simulink library "sm_wing_landing_gear_lib"  (R2015a)
settings: Solver=ode45  StartTime=0.0  StopTime=10.0  RelTol=1e-3
undefined symbols (not defined in the file): dgrey, rho_alum, X, Y, Z
libraries: sm_lib x126, sm_wing_landing_gear_lib x1
(part 1 of 4)
Description:
  | Copyright 2008-2015 The MathWorks, Inc.
settings Model: Creator=MathWorks  LastModifiedBy=batserve
settings DataIOCC: SignalLoggingSaveFormat=ModelDataLogs
settings OptimizationCC: ExpressionDepthLimit=2147483647
settings DebuggingCC: UnderspecifiedInitializationDetection=Classic  MergeDetectMultiDrivingBlocksExec=none  SolverPrmCheckMsg=warning  FcnCallInpInsideContextMsg=EnableAllAsWarning  StateNameClashWarn=warning

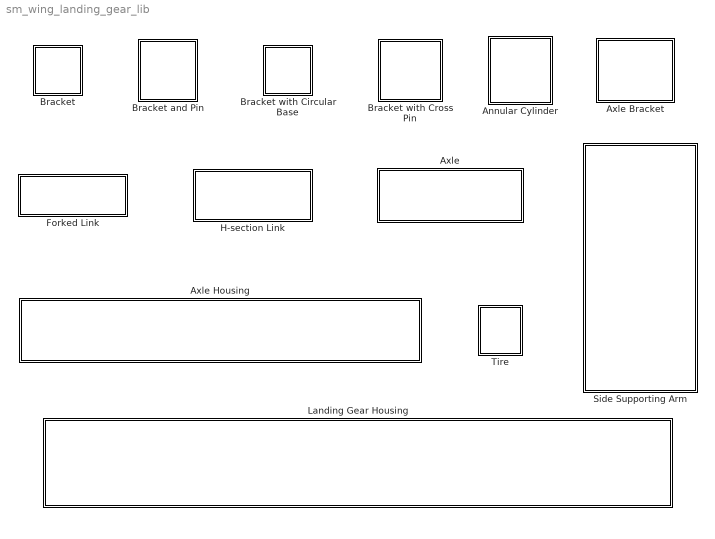
== system sm_wing_landing_gear_lib ==
  Annular Cylinder : Subsystem  mask(Annular Cylinder){Ro=10, Ri=5, L=1, rho=1000, clr=[0.5 0.5 0.5], opc=1}
      mask prompts: Ro "Cylinder outer radius (cm)"; Ri "Cylinder inner radius (cm)"; L "Cylinder length (cm)"; rho "Density (kg/m^3)"; clr "Color"; opc "Opacity"
      mask init:
      | theta = (270:-1:90)*pi/180;
      | t_semi_annular_sec = [Ri*cos(theta') Ri*sin(theta')];
      | theta = (90:1:270)*pi/180;
      | t_semi_annular_sec = [t_semi_annular_sec; Ro*cos(theta') Ro*sin(theta')];
      | b_semi_annular_sec = [-t_semi_annular_sec(end:-1:1,1) t_semi_annular_sec(end:-1:1,2)];
      mask Display:
      | image(imread('sm_wlandgear_acyl.png'));
      | port_label('RConn',1,'T')
      | port_label('LConn',1,'B')
  Axle : Subsystem  mask(Axle){Ra=4, Wd=50, Rr=20, Tr=15, rho=1000, clr=[0.5 0.5 0.5]}
      mask prompts: Ra "Axle radius (cm)"; Wd "Wheel distance (cm)"; Rr "Rim radius (cm)"; Tr "Rim thickness (cm)"; rho "Density (kg/m^3)"; clr "Color"
      mask Display:
      | image(imread('sm_wlandgear_axle.png'));
      | port_label('LConn',1,'M');
      | port_label('RConn',1,'L');
      | port_label('RConn',2,'R');
  Axle Bracket : Subsystem  mask(Axle Bracket){Wb=24, Lb=30, Tb=4, Cs=4, Rf=8, Tf=4, Rh=4, Oh=14, rho=rho_alum, clr=dgrey}
      mask prompts: Wb "Base width (cm)"; Lb "Base length (cm)"; Tb "Base thickness (cm)"; Cs "Swivel clearance (cm)"; Rf "Flange curvature radius (cm)"; Tf "Flange thickness (cm)"; Rh "Hole radius (cm)"; Oh "Hole offset (cm)"; rho "Density (kg/m^3)"; clr "Color"
      mask init:
      | hinge_sec_a = [-Lb/2 0; -Lb/2 -Cs];
      | Hp = sqrt(Oh^2 + (Lb^2)/4);
      | th = ( pi - acos(Rf/Hp) - acos(Oh/Hp) )*180/pi;
      | theta = linspace(-90-th,-90,25)*pi/180;
      | hinge_sec_a = [hinge_sec_a; Rf*cos(theta') Rf*sin(theta')-Oh];
      | theta = linspace(-90,-270,50)*pi/180;
      | hinge_sec_a = [hinge_sec_a; Rh*cos(theta') Rh*sin(theta')-Oh; 0 0];
      | hinge_sec_b = flipud([-hinge_sec_a(:,1) hinge_sec_a(:,2)]);
      mask Display:
      | image(imread('sm_wlandgear_axlebrac.png'));
      | port_label('LConn',1,'T');
      | port_label('RConn',1,'H');
  Axle Housing : Subsystem  mask(Axle Housing){L=100, W=12, T=12, Rp=4, Lp=8, r=4, La=45, Lb=10, Tb=3, Gb=3, Ro=5, Rh=2, Oh=7, rho=1000, clr=[0.5 0.5 0.5]}
      mask prompts: L "Housing length (cm)"; W "Housing width (cm)"; T "Housing thickness (cm)"; Rp "Peg radius (cm)"; Lp "Peg length (cm)"; r "Axle radius (cm)"; La "Articulating link bracket offset (cm)"; Lb "Length of bracket base (cm)"; Tb "Thickness of each bracket (cm)"; Gb "Gap between brackets (cm)"; Ro "Outer radius of bracket (cm)"; Rh "Hole radius (cm)"; Oh "Hole offset from base (cm)"; rho "Density (kg/m^3)"; clr "Color"
      mask init:
      | % Main link cross-section
      | top_xsec = [L/2 W/2; -L/2 W/2];
      | theta = (90:-1:-90)*pi/180;
      | left_semi_hole_xsec = [-L/2+r*cos(theta') r*sin(theta')];
      | bottom_xsec = [-L/2 -W/2; L/2 -W/2];
      | theta = (270:-1:90)*pi/180;
      | right_semi_hole_xsec = [L/2+r*cos(theta') r*sin(theta')];
      | link_x_section = [ top_xsec; left_semi_hole_xsec; ...
      |                    bottom_xsec; right_semi_hole_xsec];
      | 
      | % Left end cap cross-section
      | theta = (90:1:270)*pi/180;
      | outer_xsec = [(W/2)*cos(theta') (W/2)*sin(theta')];
      | theta = (270:-1:90)*pi/180;
      | inner_xsec = [r*cos(theta') r*sin(theta')];
      | left_end_x_section = [outer_xsec; inner_xsec];
      | 
      | % Right end cap cross-section
      | right_end_x_section = flipud(left_end_x_section);
      | right_end_x_section = [-right_end_x_section(:,1) right_end_x_section(:,2)];
      mask Display:
      | image(imread('sm_wlandgear_axlehouse.png'));
      | port_label('LConn',1,'FB');
      | port_label('LConn',2,'H');
      | port_label('LConn',3,'RB');
      | port_label('RConn',1,'FA');
      | port_label('RConn',2,'RA');
  Bracket : Subsystem  mask(Bracket){L=20, Tf=2, Gf=3, Ro=7, Wf=6, Ri=3, rho=1000, clr=[0.5 0.5 0.5]}
      mask prompts: L "Length of bracket base (cm)"; Tf "Thickness of each bracket (cm)"; Gf "Gap between brackets (cm)"; Ro "Outer radius of bracket (cm)"; Wf "Hole offset from base (cm)"; Ri "Hole radius (cm)"; rho "Density (kg/m^3)"; clr "Color"
      mask init:
      | flange_sec_a = [0 -L/2; Wf L/2-2*Ro];
      | theta = (-90:-1:-270)*pi/180;
      | flange_sec_a = [flange_sec_a; Ri*cos(theta')+Wf Ri*sin(theta')+L/2-Ro];
      | flange_sec_a = [flange_sec_a; Wf L/2; 0 L/2];
      | theta = (-90:1:90)*pi/180;
      | flange_sec_b = [Ro*cos(theta') Ro*sin(theta')];
      | theta = (90:-1:-90)*pi/180;
      | flange_sec_b = [flange_sec_b; Ri*cos(theta') Ri*sin(theta')];
      mask Display:
      | image(imread('sm_wlandgear_brac.png'));
      | port_label('LConn',1,'B');
      | port_label('RConn',1,'H');
  Bracket and Pin : Subsystem  mask(Bracket and Pin){Wb=6, Tb=2, L=12, Rb=12, Ro=4, Wf=5, Ri=2, Lp=14, rho=1000, clr=[0.5 0.5 0.5]}
      mask prompts: Wb "Base width (cm)"; Tb "Base thickness (cm)"; L "Base length (cm)"; Rb "Radius of curvature of bottom face (cm)"; Ro "Bracket outer radius (cm)"; Wf "Pin offset from base (cm)"; Ri "Pin radius (cm)"; Lp "Length of pin (cm)"; rho "Density (kg/m^3)"; clr "Color"
      mask help: This bracket has a curved base that can mate onto a cylindrical surface.
      mask init:
      | ang = asin(Wb/(2*Rb))*180/pi;
      | theta = (ang:-1:-ang)*pi/180;
      | base_sec = [Tb -Wb/2; Tb Wb/2; Rb*cos(theta')-Rb Rb*sin(theta')];
      | flange_sec_a = [0 -L/2; Wf L/2-2*Ro];
      | theta = (-90:-1:-270)*pi/180;
      | flange_sec_a = [flange_sec_a; Ri*cos(theta')+Wf Ri*sin(theta')+L/2-Ro];
      | flange_sec_a = [flange_sec_a; Wf L/2; 0 L/2];
      | theta = (-90:1:90)*pi/180;
      | flange_sec_b = [Ro*cos(theta') Ro*sin(theta')];
      | theta = (90:-1:-90)*pi/180;
      | flange_sec_b = [flange_sec_b; Ri*cos(theta') Ri*sin(theta')];
      mask Display:
      | image(imread('sm_wlandgear_bracketpin.png'));
      | port_label('RConn',1,'H')
      | port_label('LConn',1,'B')
  Bracket with Circular Base : Subsystem  mask(Bracket with Circular Base){Rb=12, Tb=6, Wf=22, Tf=6, Rh=5, Oh=9, rho=1000, clr=[0.5 0.5 0.5]}
      mask prompts: Rb "Base radius"; Tb "Base thickness"; Wf "Bracket width"; Tf "Bracket thickness"; Rh "Hole radius"; Oh "Hole offset"; rho "Density"; clr "Color"
      mask init:
      | flange_lower_sec = [Wf/2 0; Wf/2 Oh];
      | theta = (0:-1:-180)*pi/180;
      | x = Rh*cos(theta');
      | y = Oh + Rh*sin(theta');
      | flange_lower_sec = [flange_lower_sec; [x y]];
      | flange_lower_sec = [flange_lower_sec; -Wf/2 Oh; -Wf/2 0];
      | 
      | theta = (0:1:180)*pi/180;
      | x = (Wf/2)*cos(theta');
      | y = (Wf/2)*sin(theta');
      | flange_upper_sec = [x y];
      | theta = (180:-1:0)*pi/180;
      | x = Rh*cos(theta');
      | y = Rh*sin(theta');
      | flange_upper_sec = [flange_upper_sec; [x y]];
      mask Display:
      | image(imread('sm_wlandgear_cbbrac.png'));
      | port_label('LConn',1,'B');
      | port_label('RConn',1,'H');
  Bracket with Cross Pin : Subsystem  mask(Bracket with Cross Pin){Lb=20, Tb=3, Gb=5, Ro=7, Ri=4, Oh=14, Rp=4, Lh=40, Ohp=10, Lv=20, Ov=10, rho=1000, bclr=[0.5 0.5 0.5], pclr=[0.5 0.5 0.5]}
      mask prompts: Lb "Length of bracket base (cm)"; Tb "Thickness of each bracket (cm)"; Gb "Gap between brackets (cm)"; Ro "Radius of curvature of bracket outer surface (cm)"; Ri "Hole radius (cm)"; Oh "Hole offset from base (cm)"; Rp "Radius of pins (cm)"; Lh "Horizontal pin length (cm)"; Ohp "Hinge point offwet from center (cm)"; Lv "Vertical pin length (cm)"; Ov "Vertical pin offset from center (cm)"; rho "Density (kg/m^3)"; bclr "Bracket color"; pclr "Cross pin color"
      mask Display:
      | image(imread('sm_wlandgear_bracXpin.png'));
      | port_label('LConn',1,'P');
      | port_label('RConn',1,'B');
  Forked Link : Subsystem  mask(Forked Link){L1=72.5, L2=20, L3=11, L4=15, L5=10, L6=4, H1=16, H2=10, H3=1, H4=5, T=12, rho=1000, clr=[0.5 0.5 0.5]}
      mask prompts: L1 "L1 (cm)"; L2 "L2 (cm)"; L3 "L3 (cm)"; L4 "L4 (cm)"; L5 "L5 (cm)"; L6 "L6 (cm)"; H1 "H1 (cm)"; H2 "H2 (cm)"; H3 "H3 (cm)"; H4 "H4 (cm)"; T "T (cm)"; rho "Density (kg/m^3)"; clr "Color"
      mask help: Click on Help for the diagram illustrating the various dimensions.
      mask init:
      | cross_sec_a = [-L3 -H2/2;
      |                L6 -H2/2;
      |                (L1-L3-L4-L5) -H3/2;
      |                (L1-L3-L4-L5) 0;
      |                (L1-L3) 0;
      |                (L1-L3) -H4/2;
      |                (L1-L3-L5) -H4/2;
      |                (L2-L3) -H1/2;
      |                -L3 -H1/2];
      | cross_sec_a = flipud(cross_sec_a);           
      | cross_sec_b = flipud([cross_sec_a(:,1) -cross_sec_a(:,2)]);
      mask Help: web(fullfile(matlabroot,'toolbox','physmod','sm','smdemos','wing_landing_gear','demohelp','forkedlink.html'));
      mask Display:
      | image(imread('sm_wlandgear_forkedlink.png'));
      | port_label('LConn',1,'B');
      | port_label('RConn',1,'F');
  H-section Link : Subsystem  mask(H-section Link){Lb=5, Wb=22, Tb=12, Tf=3, Oh=25.5, Ri=4, rho=1000, clr=[0.5 0.5 0.5]}
      mask prompts: Lb "Length of base link (cm)"; Wb "Width of base link (cm)"; Tb "Thickness of base link (cm)"; Tf "Thickness of bracket (cm)"; Oh "Hole offset along bracket (cm)"; Ri "Hole radius (cm)"; rho "Density (kg/m^3)"; clr "Color"
      mask init:
      | flange_sec_a = [0 -Tb/2; Oh -Tb/2];
      | theta = (-90:-1:-270)*pi/180;
      | flange_sec_a = [flange_sec_a; Ri*cos(theta')+Oh Ri*sin(theta')];
      | flange_sec_a = [flange_sec_a; Oh Tb/2; 0 Tb/2];
      | theta = (-90:1:90)*pi/180;
      | flange_sec_b = [Tb/2*cos(theta') Tb/2*sin(theta')];
      | theta = (90:-1:-90)*pi/180;
      | flange_sec_b = [flange_sec_b; Ri*cos(theta') Ri*sin(theta')];
      mask Display:
      | image(imread('sm_wlandgear_hlink.png'));
      | port_label('LConn',1,'B');
      | port_label('RConn',1,'F');
  Landing Gear Housing : Subsystem  mask(Landing Gear Housing){L1=100, L2=60, L3=90, L4=60, L5=70, L6=30, L7=100, L8=100, T=10, H=100, Hb=75, H1=[105 -5 3*60/8-20], H2=[20 20 0], H3=[145 40 0], H4=[-10 40 0], clr=[0 0.4 0.9], Op=0.5}
      mask prompts: L1 "L1 (cm)"; L2 "L2 (cm)"; L3 "L3 (cm)"; L4 "L4 (cm)"; L5 "L5 (cm)"; L6 "L6 (cm)"; L7 "L7 (cm)"; L8 "L8 (cm)"; T "T (cm)"; H "H (cm)"; Hb "Hb (cm)"; H1 "H1 (cm)"; clr "Color"; Op "Opacity"
      mask help: Click on Help for diagram illustrating the dimensions.
      mask init:
      | wall_cross_sec_a = [0 -T/2; L1+T/2 -T/2; L1+T/2 L2-T/2; 
      |                L1+L3-T/2 L2-T/2; L1+L3-T/2 -T/2;
      |                L1+L3+L5+T/2 -T/2; L1+L3+L5+T/2 L6-T/2;
      |                L1+L3+L5+L7-T/2 L6-T/2; L1+L3+L5+L7-T/2 L6+T/2-L8;
      |                L1+L3+L5+L7+T/2 L6+T/2-L8;
      |                L1+L3+L5+L7+T/2  L6+T/2;
      |                L1+L3+L5-T/2 L6+T/2;
      |                L1+L3+L5-T/2 T/2;
      |                L1+L3+T/2 T/2;
      |                L1+L3+T/2 L4+T/2;
      |                L1-T/2 L2+T/2;
      |                L1-T/2 T/2;
      |                0 T/2];
      mask Help: web(fullfile(matlabroot,'toolbox','physmod','sm','smdemos','wing_landing_gear','demohelp','lgearhousing.html'));
      mask Display:
      | image(imread('sm_wlandgear_wall.png'));
      | port_label('LConn',1,'W');
      | port_label('RConn',1,'H1');
      | port_label('RConn',2,'H2');
      | port_label('RConn',3,'H3');
      | port_label('RConn',4,'H4');
  Side Supporting Arm : Subsystem  mask(Side Supporting Bar){L=84, W=30, H=12, T=6, Tt=9, Tb=16, Tf=2, Rf=12, Th=4, Oh=9, Rh=3, rho=rho_alum, clr=dgrey}
      mask prompts: L "L (cm)"; W "W (cm)"; H "H (cm)"; T "T (cm)"; Tt "Tt (cm)"; Tb "Tb (cm)"; Tf "Tf (cm)"; Rf "Rf (cm)"; Th "Th (cm)"; Oh "Oh (cm)"; Rh "Rh (cm)"; rho "Density"; clr "Color"
      mask help:
      | This is the side supporting arm of the landing gear. The Dimensions of the part can be set below.
      |
      | Click help for a drawing illustrating the various dimensions of the part.
      mask init:
      | th = atan(W/(L-T));
      | L1 = L-T-Tb/2;
      | slant_bar_sec = [0 -Tb/2; W L1; W-Tt L1; 0 Tb/2];
      | 
      | th = asin(H/(2*Rf))*180/pi;
      | theta = (90+th:-1:90-th)*pi/180;
      | flush_sec = [Rf*cos(theta') Rf*sin(theta')-Rf; H/2 Tf; -H/2 Tf];
      | 
      | flange_lower_sec = [H/2 0; H/2 Oh];
      | theta = (0:-1:-180)*pi/180;
      | x = Rh*cos(theta');
      | y = Oh + Rh*sin(theta');
      | flange_lower_sec = [flange_lower_sec; [x y]];
      | flange_lower_sec = [flange_lower_sec; -H/2 Oh; -H/2 0];
      | 
      | theta = (0:1:180)*pi/180;
      | x = (H/2)*cos(theta');
      | y = (H/2)*sin(theta');
      | flange_upper_sec = [x y];
      | theta = (180:-1:0)*pi/180;
      | x = Rh*cos(theta');
      | y = Rh*sin(theta');
      | flange_upper_sec = [flange_upper_sec; [x y]];
      mask Help: web(fullfile(matlabroot,'toolbox','physmod','sm','smdemos','wing_landing_gear','demohelp','sidesupportbar.html'));
      mask Display:
      | image(imread('sm_wlandgear_sidebar.png'));
      | port_label('LConn',1,'B');
      | port_label('RConn',1,'H');
  Tire : Subsystem  mask(Tire){Rt=30, Rr=20, Tt=25, rho=1000, clr=[0.5 0.5 0.5]}
      mask prompts: Rt "Tire radius (cm)"; Rr "Rim radius (cm)"; Tt "Tire thickness (cm)"; rho "Density (kg/m^3)"; clr "Color"
      mask init:
      | theta = [(0:1:359) 0]'*pi/180;
      | unit_circle = [cos(theta), sin(theta)];
      | tire_sec = [Rt * unit_circle; Rr * flipud(unit_circle)];
      mask Display:
      | image(imread('sm_wlandgear_tire.png'));
      | port_label('LConn',1,'C');

== system sm_wing_landing_gear_lib/Annular Cylinder ==
  Bottom Transform : sm_lib/Frames and Transforms/Rigid Transform  TranslationMethod=StandardAxis  TranslationLengthUnit=cm  TranslationStandardAxis=-Z  TranslationStandardOffset=L/2  TranslationCartesianOffset=[0 0 0]  TranslationROffset=0  TranslationROffsetUnits=m  TranslationZOffset=0  TranslationZOffsetUnits=m  TranslationThetaOffset=0  TranslationThetaOffsetUnits=deg  RotationMethod=None  RotationAngleUnits=deg  RotationStandardAxis=+Z  RotationAngle=0  RotationArbitraryAxis=[0 0 1]  FollAlignAxisA=+X  BaseAlignAxisA=+Y  FollAlignAxisB=+Y  BaseAlignAxisB=+Z  RotationMatrix=[1 0 0; 0 1 0; 0 0 1]  BlockFunction=simmechanics.library.frames_transforms.rigid_transform
  Left Semi Annular Cylinder : sm_lib/Body Elements/Solid  InertiaType=CalculateFromGeometry  Mass=1  MassUnits=kg  CenterOfMass=[0 0 0]  CenterOfMassUnits=m  MomentsOfInertia=[1 1 1]  MomentsOfInertiaUnits=kg*m^2  ProductsOfInertia=[0 0 0]  ProductsOfInertiaUnits=kg*m^2  DensityBased=on  Density=rho  DensityUnits=kg/(m^3)  GraphicType=FromGeometry  MarkerShape=Sphere  MarkerSize=10  MarkerSizeUnits=m  GraphicVisPropType=SimpleVisualProperties  GraphicDiffuseColor=clr  GraphicSpecularColor=[0.5 0.5 0.5 1.0]  GraphicAmbientColor=[0.5 0.0 0.0 1.0]  GraphicEmissiveColor=[0.0 0.0 0.0 1.0]  GraphicShininess=75  GraphicOpacity=opc  GeometryShape=GeneralExtrusion  RectangleSize=[1 1]  RectangleSizeUnits=m  BrickDimensions=[1 1 1]  BrickDimensionUnits=m  CylinderRadius=1  CylinderRadiusUnits=m  CylinderLength=1  CylinderLengthUnits=m  SphereRadius=1  SphereRadiusUnits=m  EllipsoidRadii=[1 1 1]  EllipsoidRadiiUnits=m  ExtrusionCrossSection=t_semi_annular_sec  ExtrusionCrossSectionUnits=cm  ExtrusionLength=L  ExtrusionLengthUnits=cm  PolygonNumSides=3  PolygonOuterRadius=1  PolygonOuterRadiusUnits=m  ExtGeomFileType=STL  ExtGeomFileUnits=m  RevolutionCrossSection=[1 1; 1 -1; 2 -1; 2 1]  RevolutionCrossSectionUnits=m  RevolutionExtent=Full  RevolutionAngle=180  RevolutionAngleUnits=deg  BlockFunction=simmechanics.library.body_elements.solid
  Right Semi Annular Cylinder : sm_lib/Body Elements/Solid  InertiaType=CalculateFromGeometry  Mass=1  MassUnits=kg  CenterOfMass=[0 0 0]  CenterOfMassUnits=m  MomentsOfInertia=[1 1 1]  MomentsOfInertiaUnits=kg*m^2  ProductsOfInertia=[0 0 0]  ProductsOfInertiaUnits=kg*m^2  DensityBased=on  Density=rho  DensityUnits=kg/(m^3)  GraphicType=FromGeometry  MarkerShape=Sphere  MarkerSize=10  MarkerSizeUnits=m  GraphicVisPropType=SimpleVisualProperties  GraphicDiffuseColor=clr  GraphicSpecularColor=[0.5 0.5 0.5 1.0]  GraphicAmbientColor=[0.5 0.0 0.0 1.0]  GraphicEmissiveColor=[0.0 0.0 0.0 1.0]  GraphicShininess=75  GraphicOpacity=opc  GeometryShape=GeneralExtrusion  RectangleSize=[1 1]  RectangleSizeUnits=m  BrickDimensions=[1 1 1]  BrickDimensionUnits=m  CylinderRadius=1  CylinderRadiusUnits=m  CylinderLength=1  CylinderLengthUnits=m  SphereRadius=1  SphereRadiusUnits=m  EllipsoidRadii=[1 1 1]  EllipsoidRadiiUnits=m  ExtrusionCrossSection=b_semi_annular_sec  ExtrusionCrossSectionUnits=cm  ExtrusionLength=L  ExtrusionLengthUnits=cm  PolygonNumSides=3  PolygonOuterRadius=1  PolygonOuterRadiusUnits=m  ExtGeomFileType=STL  ExtGeomFileUnits=m  RevolutionCrossSection=[1 1; 1 -1; 2 -1; 2 1]  RevolutionCrossSectionUnits=m  RevolutionExtent=Full  RevolutionAngle=180  RevolutionAngleUnits=deg  BlockFunction=simmechanics.library.body_elements.solid
  Top Transform : sm_lib/Frames and Transforms/Rigid Transform  TranslationMethod=StandardAxis  TranslationLengthUnit=cm  TranslationStandardAxis=+Z  TranslationStandardOffset=L/2  TranslationCartesianOffset=[0 0 0]  TranslationROffset=0  TranslationROffsetUnits=m  TranslationZOffset=0  TranslationZOffsetUnits=m  TranslationThetaOffset=0  TranslationThetaOffsetUnits=deg  RotationMethod=None  RotationAngleUnits=deg  RotationStandardAxis=+Z  RotationAngle=0  RotationArbitraryAxis=[0 0 1]  FollAlignAxisA=+X  BaseAlignAxisA=+Y  FollAlignAxisB=+Y  BaseAlignAxisB=+Z  RotationMatrix=[1 0 0; 0 1 0; 0 0 1]  BlockFunction=simmechanics.library.frames_transforms.rigid_transform
  B : PMIOPort  Port=1  Side=Left
  T : PMIOPort  Port=2  Side=Right
  connections:
  Bottom Transform/LConn1 -- Right Semi Annular Cylinder/RConn1 -- Left Semi Annular Cylinder/RConn1 -- Top Transform/LConn1
  T/RConn1 -- Top Transform/RConn1
  B/RConn1 -- Bottom Transform/RConn1

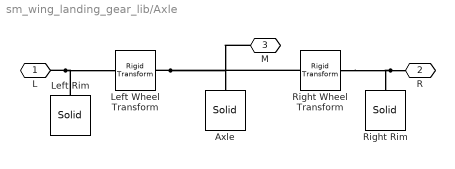
== system sm_wing_landing_gear_lib/Axle ==
  Axle : sm_lib/Body Elements/Solid  InertiaType=CalculateFromGeometry  Mass=1  MassUnits=kg  CenterOfMass=[0 0 0]  CenterOfMassUnits=m  MomentsOfInertia=[1 1 1]  MomentsOfInertiaUnits=kg*m^2  ProductsOfInertia=[0 0 0]  ProductsOfInertiaUnits=kg*m^2  DensityBased=on  Density=rho  DensityUnits=kg/(m^3)  GraphicType=FromGeometry  MarkerShape=Sphere  MarkerSize=10  MarkerSizeUnits=m  GraphicVisPropType=SimpleVisualProperties  GraphicDiffuseColor=clr  GraphicSpecularColor=[0.5 0.5 0.5 1.0]  GraphicAmbientColor=[0.5 0.0 0.0 1.0]  GraphicEmissiveColor=[0.0 0.0 0.0 1.0]  GraphicShininess=75  GraphicOpacity=1.0  GeometryShape=Cylinder  RectangleSize=[1 1]  RectangleSizeUnits=m  BrickDimensions=[1 1 1]  BrickDimensionUnits=m  CylinderRadius=Ra  CylinderRadiusUnits=cm  CylinderLength=Wd  CylinderLengthUnits=cm  SphereRadius=1  SphereRadiusUnits=m  EllipsoidRadii=[1 1 1]  EllipsoidRadiiUnits=m  ExtrusionCrossSection=[1 1; -1 1; -1 -1; 1 -1]  ExtrusionCrossSectionUnits=m  ExtrusionLength=1  ExtrusionLengthUnits=m  PolygonNumSides=3  PolygonOuterRadius=1  PolygonOuterRadiusUnits=m  ExtGeomFileType=STL  ExtGeomFileUnits=m  RevolutionCrossSection=[1 1; 1 -1; 2 -1; 2 1]  RevolutionCrossSectionUnits=m  RevolutionExtent=Full  RevolutionAngle=180  RevolutionAngleUnits=deg  BlockFunction=simmechanics.library.body_elements.solid
  "Left Rim " : sm_lib/Body Elements/Solid  InertiaType=CalculateFromGeometry  Mass=1  MassUnits=kg  CenterOfMass=[0 0 0]  CenterOfMassUnits=m  MomentsOfInertia=[1 1 1]  MomentsOfInertiaUnits=kg*m^2  ProductsOfInertia=[0 0 0]  ProductsOfInertiaUnits=kg*m^2  DensityBased=on  Density=rho  DensityUnits=kg/(m^3)  GraphicType=FromGeometry  MarkerShape=Sphere  MarkerSize=10  MarkerSizeUnits=m  GraphicVisPropType=SimpleVisualProperties  GraphicDiffuseColor=clr  GraphicSpecularColor=[0.5 0.5 0.5 1.0]  GraphicAmbientColor=[0.5 0.0 0.0 1.0]  GraphicEmissiveColor=[0.0 0.0 0.0 1.0]  GraphicShininess=75  GraphicOpacity=1.0  GeometryShape=Cylinder  RectangleSize=[1 1]  RectangleSizeUnits=m  BrickDimensions=[1 1 1]  BrickDimensionUnits=m  CylinderRadius=Rr  CylinderRadiusUnits=cm  CylinderLength=Tr  CylinderLengthUnits=cm  SphereRadius=1  SphereRadiusUnits=m  EllipsoidRadii=[1 1 1]  EllipsoidRadiiUnits=m  ExtrusionCrossSection=[1 1; -1 1; -1 -1; 1 -1]  ExtrusionCrossSectionUnits=m  ExtrusionLength=1  ExtrusionLengthUnits=m  PolygonNumSides=3  PolygonOuterRadius=1  PolygonOuterRadiusUnits=m  ExtGeomFileType=STL  ExtGeomFileUnits=m  RevolutionCrossSection=[1 1; 1 -1; 2 -1; 2 1]  RevolutionCrossSectionUnits=m  RevolutionExtent=Full  RevolutionAngle=180  RevolutionAngleUnits=deg  BlockFunction=simmechanics.library.body_elements.solid
  Left Wheel Transform : sm_lib/Frames and Transforms/Rigid Transform  TranslationMethod=StandardAxis  TranslationLengthUnit=cm  TranslationStandardAxis=-Z  TranslationStandardOffset=Wd/2 + Tr/2  TranslationCartesianOffset=[0 0 0]  TranslationROffset=0  TranslationROffsetUnits=m  TranslationZOffset=0  TranslationZOffsetUnits=m  TranslationThetaOffset=0  TranslationThetaOffsetUnits=deg  RotationMethod=None  RotationAngleUnits=deg  RotationStandardAxis=+Z  RotationAngle=0  RotationArbitraryAxis=[0 0 1]  FollAlignAxisA=+X  BaseAlignAxisA=+Y  FollAlignAxisB=+Y  BaseAlignAxisB=+Z  RotationMatrix=[1 0 0; 0 1 0; 0 0 1]  BlockFunction=simmechanics.library.frames_transforms.rigid_transform
  "Right Rim " : sm_lib/Body Elements/Solid  InertiaType=CalculateFromGeometry  Mass=1  MassUnits=kg  CenterOfMass=[0 0 0]  CenterOfMassUnits=m  MomentsOfInertia=[1 1 1]  MomentsOfInertiaUnits=kg*m^2  ProductsOfInertia=[0 0 0]  ProductsOfInertiaUnits=kg*m^2  DensityBased=on  Density=rho  DensityUnits=kg/(m^3)  GraphicType=FromGeometry  MarkerShape=Sphere  MarkerSize=10  MarkerSizeUnits=m  GraphicVisPropType=SimpleVisualProperties  GraphicDiffuseColor=clr  GraphicSpecularColor=[0.5 0.5 0.5 1.0]  GraphicAmbientColor=[0.5 0.0 0.0 1.0]  GraphicEmissiveColor=[0.0 0.0 0.0 1.0]  GraphicShininess=75  GraphicOpacity=1.0  GeometryShape=Cylinder  RectangleSize=[1 1]  RectangleSizeUnits=m  BrickDimensions=[1 1 1]  BrickDimensionUnits=m  CylinderRadius=Rr  CylinderRadiusUnits=cm  CylinderLength=Tr  CylinderLengthUnits=cm  SphereRadius=1  SphereRadiusUnits=m  EllipsoidRadii=[1 1 1]  EllipsoidRadiiUnits=m  ExtrusionCrossSection=[1 1; -1 1; -1 -1; 1 -1]  ExtrusionCrossSectionUnits=m  ExtrusionLength=1  ExtrusionLengthUnits=m  PolygonNumSides=3  PolygonOuterRadius=1  PolygonOuterRadiusUnits=m  ExtGeomFileType=STL  ExtGeomFileUnits=m  RevolutionCrossSection=[1 1; 1 -1; 2 -1; 2 1]  RevolutionCrossSectionUnits=m  RevolutionExtent=Full  RevolutionAngle=180  RevolutionAngleUnits=deg  BlockFunction=simmechanics.library.body_elements.solid
  Right Wheel Transform : sm_lib/Frames and Transforms/Rigid Transform  TranslationMethod=StandardAxis  TranslationLengthUnit=cm  TranslationStandardAxis=+Z  TranslationStandardOffset=Wd/2 + Tr/2  TranslationCartesianOffset=[0 0 0]  TranslationROffset=0  TranslationROffsetUnits=m  TranslationZOffset=0  TranslationZOffsetUnits=m  TranslationThetaOffset=0  TranslationThetaOffsetUnits=deg  RotationMethod=None  RotationAngleUnits=deg  RotationStandardAxis=+Z  RotationAngle=0  RotationArbitraryAxis=[0 0 1]  FollAlignAxisA=+X  BaseAlignAxisA=+Y  FollAlignAxisB=+Y  BaseAlignAxisB=+Z  RotationMatrix=[1 0 0; 0 1 0; 0 0 1]  BlockFunction=simmechanics.library.frames_transforms.rigid_transform
  L : PMIOPort  Port=1  Side=Right
  R : PMIOPort  Port=2  Side=Right
  M : PMIOPort  Port=3  Side=Left
  connections:
  L/RConn1 -- "Left Rim "/RConn1 -- Left Wheel Transform/RConn1
  Left Wheel Transform/LConn1 -- Right Wheel Transform/LConn1 -- Axle/RConn1 -- M/RConn1
  R/RConn1 -- Right Wheel Transform/RConn1 -- "Right Rim "/RConn1

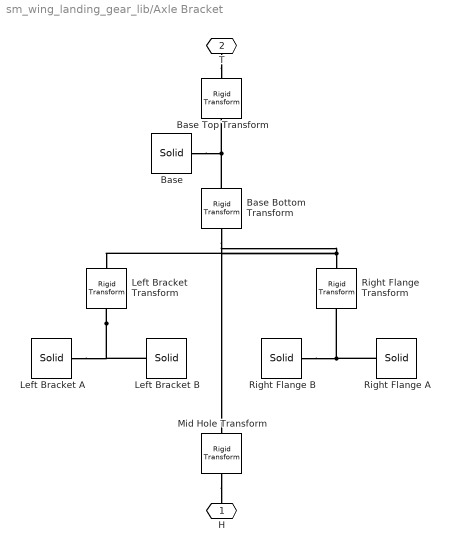
== system sm_wing_landing_gear_lib/Axle Bracket ==
  Base : sm_lib/Body Elements/Solid  InertiaType=CalculateFromGeometry  Mass=1  MassUnits=kg  CenterOfMass=[0 0 0]  CenterOfMassUnits=m  MomentsOfInertia=[1 1 1]  MomentsOfInertiaUnits=kg*m^2  ProductsOfInertia=[0 0 0]  ProductsOfInertiaUnits=kg*m^2  DensityBased=on  Density=rho  DensityUnits=kg/(m^3)  GraphicType=FromGeometry  MarkerShape=Sphere  MarkerSize=10  MarkerSizeUnits=m  GraphicVisPropType=SimpleVisualProperties  GraphicDiffuseColor=clr  GraphicSpecularColor=[0.5 0.5 0.5 1.0]  GraphicAmbientColor=[0.5 0.0 0.0 1.0]  GraphicEmissiveColor=[0.0 0.0 0.0 1.0]  GraphicShininess=75  GraphicOpacity=1.0  GeometryShape=Brick  RectangleSize=[1 1]  RectangleSizeUnits=m  BrickDimensions=[Wb Lb Tb]  BrickDimensionUnits=cm  CylinderRadius=1  CylinderRadiusUnits=m  CylinderLength=1  CylinderLengthUnits=m  SphereRadius=1  SphereRadiusUnits=m  EllipsoidRadii=[1 1 1]  EllipsoidRadiiUnits=m  ExtrusionCrossSection=[1 1; -1 1; -1 -1; 1 -1]  ExtrusionCrossSectionUnits=m  ExtrusionLength=1  ExtrusionLengthUnits=m  PolygonNumSides=3  PolygonOuterRadius=1  PolygonOuterRadiusUnits=m  ExtGeomFileType=STL  ExtGeomFileUnits=m  RevolutionCrossSection=[1 1; 1 -1; 2 -1; 2 1]  RevolutionCrossSectionUnits=m  RevolutionExtent=Full  RevolutionAngle=180  RevolutionAngleUnits=deg  BlockFunction=simmechanics.library.body_elements.solid
  Base Bottom Transform : sm_lib/Frames and Transforms/Rigid Transform  TranslationMethod=StandardAxis  TranslationLengthUnit=cm  TranslationStandardAxis=-Z  TranslationStandardOffset=Tb/2  TranslationCartesianOffset=[0 0 0]  TranslationROffset=0  TranslationROffsetUnits=m  TranslationZOffset=0  TranslationZOffsetUnits=m  TranslationThetaOffset=0  TranslationThetaOffsetUnits=deg  RotationMethod=None  RotationAngleUnits=deg  RotationStandardAxis=+Z  RotationAngle=0  RotationArbitraryAxis=[0 0 1]  FollAlignAxisA=+X  BaseAlignAxisA=+Y  FollAlignAxisB=+Y  BaseAlignAxisB=+Z  RotationMatrix=[1 0 0; 0 1 0; 0 0 1]  BlockFunction=simmechanics.library.frames_transforms.rigid_transform
  Base Top Transform : sm_lib/Frames and Transforms/Rigid Transform  TranslationMethod=StandardAxis  TranslationLengthUnit=cm  TranslationStandardAxis=+Z  TranslationStandardOffset=Tb/2  TranslationCartesianOffset=[0 0 0]  TranslationROffset=0  TranslationROffsetUnits=m  TranslationZOffset=0  TranslationZOffsetUnits=m  TranslationThetaOffset=0  TranslationThetaOffsetUnits=deg  RotationMethod=None  RotationAngleUnits=deg  RotationStandardAxis=+Z  RotationAngle=0  RotationArbitraryAxis=[0 0 1]  FollAlignAxisA=+X  BaseAlignAxisA=+Y  FollAlignAxisB=+Y  BaseAlignAxisB=+Z  RotationMatrix=[1 0 0; 0 1 0; 0 0 1]  BlockFunction=simmechanics.library.frames_transforms.rigid_transform
  Left Bracket A : sm_lib/Body Elements/Solid  InertiaType=CalculateFromGeometry  Mass=1  MassUnits=kg  CenterOfMass=[0 0 0]  CenterOfMassUnits=m  MomentsOfInertia=[1 1 1]  MomentsOfInertiaUnits=kg*m^2  ProductsOfInertia=[0 0 0]  ProductsOfInertiaUnits=kg*m^2  DensityBased=on  Density=rho  DensityUnits=kg/(m^3)  GraphicType=FromGeometry  MarkerShape=Sphere  MarkerSize=10  MarkerSizeUnits=m  GraphicVisPropType=SimpleVisualProperties  GraphicDiffuseColor=clr  GraphicSpecularColor=[0.5 0.5 0.5 1.0]  GraphicAmbientColor=[0.5 0.0 0.0 1.0]  GraphicEmissiveColor=[0.0 0.0 0.0 1.0]  GraphicShininess=75  GraphicOpacity=1.0  GeometryShape=GeneralExtrusion  RectangleSize=[1 1]  RectangleSizeUnits=m  BrickDimensions=[1 1 1]  BrickDimensionUnits=cm  CylinderRadius=1  CylinderRadiusUnits=m  CylinderLength=1  CylinderLengthUnits=m  SphereRadius=1  SphereRadiusUnits=m  EllipsoidRadii=[1 1 1]  EllipsoidRadiiUnits=m  ExtrusionCrossSection=hinge_sec_b  ExtrusionCrossSectionUnits=cm  ExtrusionLength=Tf  ExtrusionLengthUnits=cm  PolygonNumSides=3  PolygonOuterRadius=1  PolygonOuterRadiusUnits=m  ExtGeomFileType=STL  ExtGeomFileUnits=m  RevolutionCrossSection=[1 1; 1 -1; 2 -1; 2 1]  RevolutionCrossSectionUnits=m  RevolutionExtent=Full  RevolutionAngle=180  RevolutionAngleUnits=deg  BlockFunction=simmechanics.library.body_elements.solid
  Left Bracket B : sm_lib/Body Elements/Solid  InertiaType=CalculateFromGeometry  Mass=1  MassUnits=kg  CenterOfMass=[0 0 0]  CenterOfMassUnits=m  MomentsOfInertia=[1 1 1]  MomentsOfInertiaUnits=kg*m^2  ProductsOfInertia=[0 0 0]  ProductsOfInertiaUnits=kg*m^2  DensityBased=on  Density=rho  DensityUnits=kg/(m^3)  GraphicType=FromGeometry  MarkerShape=Sphere  MarkerSize=10  MarkerSizeUnits=m  GraphicVisPropType=SimpleVisualProperties  GraphicDiffuseColor=clr  GraphicSpecularColor=[0.5 0.5 0.5 1.0]  GraphicAmbientColor=[0.5 0.0 0.0 1.0]  GraphicEmissiveColor=[0.0 0.0 0.0 1.0]  GraphicShininess=75  GraphicOpacity=1.0  GeometryShape=GeneralExtrusion  RectangleSize=[1 1]  RectangleSizeUnits=m  BrickDimensions=[1 1 1]  BrickDimensionUnits=cm  CylinderRadius=1  CylinderRadiusUnits=m  CylinderLength=1  CylinderLengthUnits=m  SphereRadius=1  SphereRadiusUnits=m  EllipsoidRadii=[1 1 1]  EllipsoidRadiiUnits=m  ExtrusionCrossSection=hinge_sec_a  ExtrusionCrossSectionUnits=cm  ExtrusionLength=Tf  ExtrusionLengthUnits=cm  PolygonNumSides=3  PolygonOuterRadius=1  PolygonOuterRadiusUnits=m  ExtGeomFileType=STL  ExtGeomFileUnits=m  RevolutionCrossSection=[1 1; 1 -1; 2 -1; 2 1]  RevolutionCrossSectionUnits=m  RevolutionExtent=Full  RevolutionAngle=180  RevolutionAngleUnits=deg  BlockFunction=simmechanics.library.body_elements.solid
  Left Bracket Transform : sm_lib/Frames and Transforms/Rigid Transform  TranslationMethod=StandardAxis  TranslationLengthUnit=cm  TranslationStandardAxis=-X  TranslationStandardOffset=Wb/2 - Tf/2  TranslationCartesianOffset=[0 0 0]  TranslationROffset=0  TranslationROffsetUnits=m  TranslationZOffset=0  TranslationZOffsetUnits=m  TranslationThetaOffset=0  TranslationThetaOffsetUnits=deg  RotationMethod=AlignedAxes  RotationAngleUnits=deg  RotationStandardAxis=+Z  RotationAngle=0  RotationArbitraryAxis=[0 0 1]  FollAlignAxisA=+Z  BaseAlignAxisA=+X  FollAlignAxisB=+X  BaseAlignAxisB=+Y  RotationMatrix=[1 0 0; 0 1 0; 0 0 1]  BlockFunction=simmechanics.library.frames_transforms.rigid_transform
  Mid Hole Transform : sm_lib/Frames and Transforms/Rigid Transform  TranslationMethod=StandardAxis  TranslationLengthUnit=cm  TranslationStandardAxis=-Z  TranslationStandardOffset=Oh  TranslationCartesianOffset=[0 0 0]  TranslationROffset=0  TranslationROffsetUnits=m  TranslationZOffset=0  TranslationZOffsetUnits=m  TranslationThetaOffset=0  TranslationThetaOffsetUnits=deg  RotationMethod=AlignedAxes  RotationAngleUnits=deg  RotationStandardAxis=+Z  RotationAngle=0  RotationArbitraryAxis=[0 0 1]  FollAlignAxisA=+Z  BaseAlignAxisA=+X  FollAlignAxisB=+X  BaseAlignAxisB=+Y  RotationMatrix=[1 0 0; 0 1 0; 0 0 1]  BlockFunction=simmechanics.library.frames_transforms.rigid_transform
  Right Flange A : sm_lib/Body Elements/Solid  InertiaType=CalculateFromGeometry  Mass=1  MassUnits=kg  CenterOfMass=[0 0 0]  CenterOfMassUnits=m  MomentsOfInertia=[1 1 1]  MomentsOfInertiaUnits=kg*m^2  ProductsOfInertia=[0 0 0]  ProductsOfInertiaUnits=kg*m^2  DensityBased=on  Density=rho  DensityUnits=kg/(m^3)  GraphicType=FromGeometry  MarkerShape=Sphere  MarkerSize=10  MarkerSizeUnits=m  GraphicVisPropType=SimpleVisualProperties  GraphicDiffuseColor=clr  GraphicSpecularColor=[0.5 0.5 0.5 1.0]  GraphicAmbientColor=[0.5 0.0 0.0 1.0]  GraphicEmissiveColor=[0.0 0.0 0.0 1.0]  GraphicShininess=75  GraphicOpacity=1.0  GeometryShape=GeneralExtrusion  RectangleSize=[1 1]  RectangleSizeUnits=m  BrickDimensions=[1 1 1]  BrickDimensionUnits=cm  CylinderRadius=1  CylinderRadiusUnits=m  CylinderLength=1  CylinderLengthUnits=m  SphereRadius=1  SphereRadiusUnits=m  EllipsoidRadii=[1 1 1]  EllipsoidRadiiUnits=m  ExtrusionCrossSection=hinge_sec_a  ExtrusionCrossSectionUnits=cm  ExtrusionLength=Tf  ExtrusionLengthUnits=cm  PolygonNumSides=3  PolygonOuterRadius=1  PolygonOuterRadiusUnits=m  ExtGeomFileType=STL  ExtGeomFileUnits=m  RevolutionCrossSection=[1 1; 1 -1; 2 -1; 2 1]  RevolutionCrossSectionUnits=m  RevolutionExtent=Full  RevolutionAngle=180  RevolutionAngleUnits=deg  BlockFunction=simmechanics.library.body_elements.solid
  Right Flange B : sm_lib/Body Elements/Solid  InertiaType=CalculateFromGeometry  Mass=1  MassUnits=kg  CenterOfMass=[0 0 0]  CenterOfMassUnits=m  MomentsOfInertia=[1 1 1]  MomentsOfInertiaUnits=kg*m^2  ProductsOfInertia=[0 0 0]  ProductsOfInertiaUnits=kg*m^2  DensityBased=on  Density=rho  DensityUnits=kg/(m^3)  GraphicType=FromGeometry  MarkerShape=Sphere  MarkerSize=10  MarkerSizeUnits=m  GraphicVisPropType=SimpleVisualProperties  GraphicDiffuseColor=clr  GraphicSpecularColor=[0.5 0.5 0.5 1.0]  GraphicAmbientColor=[0.5 0.0 0.0 1.0]  GraphicEmissiveColor=[0.0 0.0 0.0 1.0]  GraphicShininess=75  GraphicOpacity=1.0  GeometryShape=GeneralExtrusion  RectangleSize=[1 1]  RectangleSizeUnits=m  BrickDimensions=[1 1 1]  BrickDimensionUnits=cm  CylinderRadius=1  CylinderRadiusUnits=m  CylinderLength=1  CylinderLengthUnits=m  SphereRadius=1  SphereRadiusUnits=m  EllipsoidRadii=[1 1 1]  EllipsoidRadiiUnits=m  ExtrusionCrossSection=hinge_sec_b  ExtrusionCrossSectionUnits=cm  ExtrusionLength=Tf  ExtrusionLengthUnits=cm  PolygonNumSides=3  PolygonOuterRadius=1  PolygonOuterRadiusUnits=m  ExtGeomFileType=STL  ExtGeomFileUnits=m  RevolutionCrossSection=[1 1; 1 -1; 2 -1; 2 1]  RevolutionCrossSectionUnits=m  RevolutionExtent=Full  RevolutionAngle=180  RevolutionAngleUnits=deg  BlockFunction=simmechanics.library.body_elements.solid
  Right Flange Transform : sm_lib/Frames and Transforms/Rigid Transform  TranslationMethod=StandardAxis  TranslationLengthUnit=cm  TranslationStandardAxis=+X  TranslationStandardOffset=Wb/2 - Tf/2  TranslationCartesianOffset=[0 0 0]  TranslationROffset=0  TranslationROffsetUnits=m  TranslationZOffset=0  TranslationZOffsetUnits=m  TranslationThetaOffset=0  TranslationThetaOffsetUnits=deg  RotationMethod=AlignedAxes  RotationAngleUnits=deg  RotationStandardAxis=+Z  RotationAngle=0  RotationArbitraryAxis=[0 0 1]  FollAlignAxisA=+Z  BaseAlignAxisA=+X  FollAlignAxisB=+X  BaseAlignAxisB=+Y  RotationMatrix=[1 0 0; 0 1 0; 0 0 1]  BlockFunction=simmechanics.library.frames_transforms.rigid_transform
  H : PMIOPort  Port=1  Side=Right
  T : PMIOPort  Port=2  Side=Left
  connections:
  T/RConn1 -- Base Top Transform/RConn1
  Base Bottom Transform/LConn1 -- Base Top Transform/LConn1 -- Base/RConn1
  Right Flange Transform/LConn1 -- Base Bottom Transform/RConn1 -- Mid Hole Transform/LConn1 -- Left Bracket Transform/LConn1
  Right Flange A/RConn1 -- Right Flange Transform/RConn1 -- Right Flange B/RConn1
  Mid Hole Transform/RConn1 -- H/RConn1
  Left Bracket Transform/RConn1 -- Left Bracket A/RConn1 -- Left Bracket B/RConn1

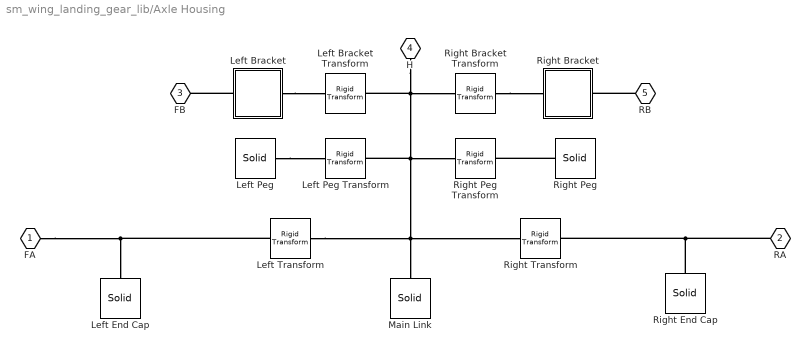
== system sm_wing_landing_gear_lib/Axle Housing ==
  Left Transform : sm_lib/Frames and Transforms/Rigid Transform  TranslationMethod=StandardAxis  TranslationLengthUnit=cm  TranslationStandardAxis=-X  TranslationStandardOffset=L/2  TranslationCartesianOffset=[0 0 0]  TranslationROffset=0  TranslationROffsetUnits=m  TranslationZOffset=0  TranslationZOffsetUnits=m  TranslationThetaOffset=0  TranslationThetaOffsetUnits=deg  RotationMethod=None  RotationAngleUnits=deg  RotationStandardAxis=+Z  RotationAngle=0  RotationArbitraryAxis=[0 0 1]  FollAlignAxisA=+X  BaseAlignAxisA=+Y  FollAlignAxisB=+Y  BaseAlignAxisB=+Z  RotationMatrix=[1 0 0; 0 1 0; 0 0 1]  BlockFunction=simmechanics.library.frames_transforms.rigid_transform
  Left Bracket : Subsystem  mask(Bracket){L=Lb, Tf=Tb, Gf=Gb, Ro=Ro, Wf=Oh, Ri=Rh, rho=rho, clr=clr}
      mask prompts: L "Length of bracket base (cm)"; Tf "Thickness of each bracket (cm)"; Gf "Gap between brackets (cm)"; Ro "Outer radius of bracket (cm)"; Wf "Hole offset from base (cm)"; Ri "Hole radius (cm)"; rho "Density (kg/m^3)"; clr "Color"
      mask init: same as sm_wing_landing_gear_lib/Bracket
      mask Display:
      | image(imread('sm_wlandgear_brac.png'));
      | port_label('LConn',1,'B');
      | port_label('RConn',1,'H');
  Left Bracket Transform : sm_lib/Frames and Transforms/Rigid Transform  TranslationMethod=Cartesian  TranslationLengthUnit=cm  TranslationStandardAxis=+Z  TranslationStandardOffset=0  TranslationCartesianOffset=[-La W/2 0]  TranslationROffset=0  TranslationROffsetUnits=m  TranslationZOffset=0  TranslationZOffsetUnits=m  TranslationThetaOffset=0  TranslationThetaOffsetUnits=deg  RotationMethod=AlignedAxes  RotationAngleUnits=deg  RotationStandardAxis=+Z  RotationAngle=0  RotationArbitraryAxis=[0 0 1]  FollAlignAxisA=+Z  BaseAlignAxisA=+X  FollAlignAxisB=+X  BaseAlignAxisB=+Y  RotationMatrix=[1 0 0; 0 1 0; 0 0 1]  BlockFunction=simmechanics.library.frames_transforms.rigid_transform
  Left End Cap : sm_lib/Body Elements/Solid  InertiaType=CalculateFromGeometry  Mass=1  MassUnits=kg  CenterOfMass=[0 0 0]  CenterOfMassUnits=m  MomentsOfInertia=[1 1 1]  MomentsOfInertiaUnits=kg*m^2  ProductsOfInertia=[0 0 0]  ProductsOfInertiaUnits=kg*m^2  DensityBased=on  Density=rho  DensityUnits=kg/m^3  GraphicType=FromGeometry  MarkerShape=Sphere  MarkerSize=1  MarkerSizeUnits=m  GraphicVisPropType=SimpleVisualProperties  GraphicDiffuseColor=clr  GraphicSpecularColor=ddgrey  GraphicAmbientColor=grey  GraphicEmissiveColor=[0.1 0.1 0.1]  GraphicShininess=24.0  GraphicOpacity=1  GeometryShape=GeneralExtrusion  RectangleSize=[1 1]  RectangleSizeUnits=m  BrickDimensions=[1 1 1]  BrickDimensionUnits=m  CylinderRadius=1  CylinderRadiusUnits=m  CylinderLength=1  CylinderLengthUnits=m  SphereRadius=1  SphereRadiusUnits=m  EllipsoidRadii=[1 1 1]  EllipsoidRadiiUnits=m  ExtrusionCrossSection=left_end_x_section  ExtrusionCrossSectionUnits=cm  ExtrusionLength=T  ExtrusionLengthUnits=cm  PolygonNumSides=1  PolygonOuterRadius=1  PolygonOuterRadiusUnits=m  ExtGeomFileType=STL  ExtGeomFileUnits=m  RevolutionCrossSection=[1 1; 1 -1; 2 -1; 2 1]  RevolutionCrossSectionUnits=m  RevolutionExtent=Full  RevolutionAngle=180  RevolutionAngleUnits=deg  BlockFunction=simmechanics.library.body_elements.solid
  Left Peg : sm_lib/Body Elements/Solid  InertiaType=CalculateFromGeometry  Mass=1  MassUnits=kg  CenterOfMass=[0 0 0]  CenterOfMassUnits=m  MomentsOfInertia=[1 1 1]  MomentsOfInertiaUnits=kg*m^2  ProductsOfInertia=[0 0 0]  ProductsOfInertiaUnits=kg*m^2  DensityBased=on  Density=rho  DensityUnits=kg/(m^3)  GraphicType=FromGeometry  MarkerShape=Sphere  MarkerSize=10  MarkerSizeUnits=m  GraphicVisPropType=SimpleVisualProperties  GraphicDiffuseColor=clr  GraphicSpecularColor=[0.5 0.5 0.5 1.0]  GraphicAmbientColor=[0.5 0.0 0.0 1.0]  GraphicEmissiveColor=[0.0 0.0 0.0 1.0]  GraphicShininess=75  GraphicOpacity=1.0  GeometryShape=Cylinder  RectangleSize=[1 1]  RectangleSizeUnits=m  BrickDimensions=[1 1 1]  BrickDimensionUnits=m  CylinderRadius=Rp  CylinderRadiusUnits=cm  CylinderLength=Lp  CylinderLengthUnits=cm  SphereRadius=1  SphereRadiusUnits=m  EllipsoidRadii=[1 1 1]  EllipsoidRadiiUnits=m  ExtrusionCrossSection=[1 1; -1 1; -1 -1; 1 -1]  ExtrusionCrossSectionUnits=m  ExtrusionLength=1  ExtrusionLengthUnits=m  PolygonNumSides=3  PolygonOuterRadius=1  PolygonOuterRadiusUnits=m  ExtGeomFileType=STL  ExtGeomFileUnits=m  RevolutionCrossSection=[1 1; 1 -1; 2 -1; 2 1]  RevolutionCrossSectionUnits=m  RevolutionExtent=Full  RevolutionAngle=180  RevolutionAngleUnits=deg  BlockFunction=simmechanics.library.body_elements.solid
  Left Peg Transform : sm_lib/Frames and Transforms/Rigid Transform  TranslationMethod=StandardAxis  TranslationLengthUnit=cm  TranslationStandardAxis=-Z  TranslationStandardOffset=T/2 + Lp/2  TranslationCartesianOffset=[0 0 0]  TranslationROffset=0  TranslationROffsetUnits=m  TranslationZOffset=0  TranslationZOffsetUnits=m  TranslationThetaOffset=0  TranslationThetaOffsetUnits=deg  RotationMethod=None  RotationAngleUnits=deg  RotationStandardAxis=+Z  RotationAngle=0  RotationArbitraryAxis=[0 0 1]  FollAlignAxisA=+X  BaseAlignAxisA=+Y  FollAlignAxisB=+Y  BaseAlignAxisB=+Z  RotationMatrix=[1 0 0; 0 1 0; 0 0 1]  BlockFunction=simmechanics.library.frames_transforms.rigid_transform
  Main Link : sm_lib/Body Elements/Solid  InertiaType=CalculateFromGeometry  Mass=1  MassUnits=kg  CenterOfMass=[0 0 0]  CenterOfMassUnits=m  MomentsOfInertia=[1 1 1]  MomentsOfInertiaUnits=kg*m^2  ProductsOfInertia=[0 0 0]  ProductsOfInertiaUnits=kg*m^2  DensityBased=on  Density=rho  DensityUnits=kg/m^3  GraphicType=FromGeometry  MarkerShape=Sphere  MarkerSize=1  MarkerSizeUnits=m  GraphicVisPropType=SimpleVisualProperties  GraphicDiffuseColor=clr  GraphicSpecularColor=ddgrey  GraphicAmbientColor=grey  GraphicEmissiveColor=[0.1 0.1 0.1]  GraphicShininess=24.0  GraphicOpacity=1  GeometryShape=GeneralExtrusion  RectangleSize=[1 1]  RectangleSizeUnits=m  BrickDimensions=[1 1 1]  BrickDimensionUnits=m  CylinderRadius=1  CylinderRadiusUnits=m  CylinderLength=1  CylinderLengthUnits=m  SphereRadius=1  SphereRadiusUnits=m  EllipsoidRadii=[1 1 1]  EllipsoidRadiiUnits=m  ExtrusionCrossSection=link_x_section  ExtrusionCrossSectionUnits=cm  ExtrusionLength=T  ExtrusionLengthUnits=cm  PolygonNumSides=1  PolygonOuterRadius=1  PolygonOuterRadiusUnits=m  ExtGeomFileType=STL  ExtGeomFileUnits=m  RevolutionCrossSection=[1 1; 1 -1; 2 -1; 2 1]  RevolutionCrossSectionUnits=m  RevolutionExtent=Full  RevolutionAngle=180  RevolutionAngleUnits=deg  BlockFunction=simmechanics.library.body_elements.solid
  Right Transform : sm_lib/Frames and Transforms/Rigid Transform  TranslationMethod=StandardAxis  TranslationLengthUnit=cm  TranslationStandardAxis=+X  TranslationStandardOffset=L/2  TranslationCartesianOffset=[0 0 0]  TranslationROffset=0  TranslationROffsetUnits=m  TranslationZOffset=0  TranslationZOffsetUnits=m  TranslationThetaOffset=0  TranslationThetaOffsetUnits=deg  RotationMethod=None  RotationAngleUnits=deg  RotationStandardAxis=+Z  RotationAngle=0  RotationArbitraryAxis=[0 0 1]  FollAlignAxisA=+X  BaseAlignAxisA=+Y  FollAlignAxisB=+Y  BaseAlignAxisB=+Z  RotationMatrix=[1 0 0; 0 1 0; 0 0 1]  BlockFunction=simmechanics.library.frames_transforms.rigid_transform
  Right Bracket : Subsystem  mask(Bracket){L=Lb, Tf=Tb, Gf=Gb, Ro=Ro, Wf=Oh, Ri=Rh, rho=rho, clr=clr}
      mask prompts: L "Length of bracket base (cm)"; Tf "Thickness of each bracket (cm)"; Gf "Gap between brackets (cm)"; Ro "Outer radius of bracket (cm)"; Wf "Hole offset from base (cm)"; Ri "Hole radius (cm)"; rho "Density (kg/m^3)"; clr "Color"
      mask init: same as sm_wing_landing_gear_lib/Bracket
      mask Display:
      | image(imread('sm_wlandgear_brac.png'));
      | port_label('LConn',1,'B');
      | port_label('RConn',1,'H');
  Right Bracket Transform : sm_lib/Frames and Transforms/Rigid Transform  TranslationMethod=Cartesian  TranslationLengthUnit=cm  TranslationStandardAxis=+Z  TranslationStandardOffset=0  TranslationCartesianOffset=[La W/2 0]  TranslationROffset=0  TranslationROffsetUnits=m  TranslationZOffset=0  TranslationZOffsetUnits=m  TranslationThetaOffset=0  TranslationThetaOffsetUnits=deg  RotationMethod=AlignedAxes  RotationAngleUnits=deg  RotationStandardAxis=+Z  RotationAngle=0  RotationArbitraryAxis=[0 0 1]  FollAlignAxisA=+Z  BaseAlignAxisA=-X  FollAlignAxisB=+X  BaseAlignAxisB=+Y  RotationMatrix=[1 0 0; 0 1 0; 0 0 1]  BlockFunction=simmechanics.library.frames_transforms.rigid_transform
  Right End Cap : sm_lib/Body Elements/Solid  InertiaType=CalculateFromGeometry  Mass=1  MassUnits=kg  CenterOfMass=[0 0 0]  CenterOfMassUnits=m  MomentsOfInertia=[1 1 1]  MomentsOfInertiaUnits=kg*m^2  ProductsOfInertia=[0 0 0]  ProductsOfInertiaUnits=kg*m^2  DensityBased=on  Density=rho  DensityUnits=kg/m^3  GraphicType=FromGeometry  MarkerShape=Sphere  MarkerSize=1  MarkerSizeUnits=m  GraphicVisPropType=SimpleVisualProperties  GraphicDiffuseColor=clr  GraphicSpecularColor=ddgrey  GraphicAmbientColor=grey  GraphicEmissiveColor=[0.1 0.1 0.1]  GraphicShininess=24.0  GraphicOpacity=1  GeometryShape=GeneralExtrusion  RectangleSize=[1 1]  RectangleSizeUnits=m  BrickDimensions=[1 1 1]  BrickDimensionUnits=m  CylinderRadius=1  CylinderRadiusUnits=m  CylinderLength=1  CylinderLengthUnits=m  SphereRadius=1  SphereRadiusUnits=m  EllipsoidRadii=[1 1 1]  EllipsoidRadiiUnits=m  ExtrusionCrossSection=right_end_x_section  ExtrusionCrossSectionUnits=cm  ExtrusionLength=T  ExtrusionLengthUnits=cm  PolygonNumSides=1  PolygonOuterRadius=1  PolygonOuterRadiusUnits=m  ExtGeomFileType=STL  ExtGeomFileUnits=m  RevolutionCrossSection=[1 1; 1 -1; 2 -1; 2 1]  RevolutionCrossSectionUnits=m  RevolutionExtent=Full  RevolutionAngle=180  RevolutionAngleUnits=deg  BlockFunction=simmechanics.library.body_elements.solid
  Right Peg : sm_lib/Body Elements/Solid  InertiaType=CalculateFromGeometry  Mass=1  MassUnits=kg  CenterOfMass=[0 0 0]  CenterOfMassUnits=m  MomentsOfInertia=[1 1 1]  MomentsOfInertiaUnits=kg*m^2  ProductsOfInertia=[0 0 0]  ProductsOfInertiaUnits=kg*m^2  DensityBased=on  Density=rho  DensityUnits=kg/(m^3)  GraphicType=FromGeometry  MarkerShape=Sphere  MarkerSize=10  MarkerSizeUnits=m  GraphicVisPropType=SimpleVisualProperties  GraphicDiffuseColor=clr  GraphicSpecularColor=[0.5 0.5 0.5 1.0]  GraphicAmbientColor=[0.5 0.0 0.0 1.0]  GraphicEmissiveColor=[0.0 0.0 0.0 1.0]  GraphicShininess=75  GraphicOpacity=1.0  GeometryShape=Cylinder  RectangleSize=[1 1]  RectangleSizeUnits=m  BrickDimensions=[1 1 1]  BrickDimensionUnits=m  CylinderRadius=Rp  CylinderRadiusUnits=cm  CylinderLength=Lp  CylinderLengthUnits=cm  SphereRadius=1  SphereRadiusUnits=m  EllipsoidRadii=[1 1 1]  EllipsoidRadiiUnits=m  ExtrusionCrossSection=[1 1; -1 1; -1 -1; 1 -1]  ExtrusionCrossSectionUnits=m  ExtrusionLength=1  ExtrusionLengthUnits=m  PolygonNumSides=3  PolygonOuterRadius=1  PolygonOuterRadiusUnits=m  ExtGeomFileType=STL  ExtGeomFileUnits=m  RevolutionCrossSection=[1 1; 1 -1; 2 -1; 2 1]  RevolutionCrossSectionUnits=m  RevolutionExtent=Full  RevolutionAngle=180  RevolutionAngleUnits=deg  BlockFunction=simmechanics.library.body_elements.solid
  Right Peg Transform : sm_lib/Frames and Transforms/Rigid Transform  TranslationMethod=StandardAxis  TranslationLengthUnit=cm  TranslationStandardAxis=+Z  TranslationStandardOffset=T/2 + Lp/2  TranslationCartesianOffset=[0 0 0]  TranslationROffset=0  TranslationROffsetUnits=m  TranslationZOffset=0  TranslationZOffsetUnits=m  TranslationThetaOffset=0  TranslationThetaOffsetUnits=deg  RotationMethod=None  RotationAngleUnits=deg  RotationStandardAxis=+Z  RotationAngle=0  RotationArbitraryAxis=[0 0 1]  FollAlignAxisA=+X  BaseAlignAxisA=+Y  FollAlignAxisB=+Y  BaseAlignAxisB=+Z  RotationMatrix=[1 0 0; 0 1 0; 0 0 1]  BlockFunction=simmechanics.library.frames_transforms.rigid_transform
  FA : PMIOPort  Port=1  Side=Right
  RA : PMIOPort  Port=2  Side=Right
  FB : PMIOPort  Port=3  Side=Left
  H : PMIOPort  Port=4  Side=Left
  RB : PMIOPort  Port=5  Side=Left
  connections:
  H/RConn1 -- Left Transform/LConn1 -- Main Link/RConn1 -- Right Transform/LConn1 -- Right Peg Transform/LConn1 -- Left Peg Transform/LConn1 -- Right Bracket Transform/LConn1 -- Left Bracket Transform/LConn1
  FA/RConn1 -- Left Transform/RConn1 -- Left End Cap/RConn1
  RA/RConn1 -- Right Transform/RConn1 -- Right End Cap/RConn1
  Left Peg/RConn1 -- Left Peg Transform/RConn1
  Right Peg/RConn1 -- Right Peg Transform/RConn1
  Right Bracket Transform/RConn1 -- Right Bracket/LConn1
  RB/RConn1 -- Right Bracket/RConn1
  Left Bracket/RConn1 -- FB/RConn1
  Left Bracket/LConn1 -- Left Bracket Transform/RConn1
